simulink model "MotorCtrl_DTC_Math"  (R2023b)
settings: Solver=FixedStepDiscrete  StartTime=0.0  StopTime=5  FixedStep=MC_Sim_BaseStep  RelTol=1e-3  EnableMultiTasking=on
values from neighbouring files (symbols this model uses):
  MC_ADC_BitNum = 0.0    [MotorControlDataDictionary_Math.sldd]
  MC_ADC_Offset = 0.0    [MotorControlDataDictionary_Math.sldd]
  MC_ADC_VRef = 1.0    [MotorControlDataDictionary_Math.sldd]
  MC_Const_DutyL = 0.2    [MotorControlDataDictionary_Math.sldd]
  MC_Const_DutyS = 0.8    [MotorControlDataDictionary_Math.sldd]
  MC_CSA_Gain = 1.0    [MotorControlDataDictionary_Math.sldd]
  MC_Input_Vdc = 13.5    [MotorControlDataDictionary_Math.sldd]
  MC_MOS_DeadTime = 1.0E-6    [MotorControlDataDictionary_Math.sldd]
  MC_Motor_Mechinal_Damp = 1.0E-5    [MotorControlDataDictionary_Math.sldd]
  MC_Motor_Mechinal_Fric = 0.0    [MotorControlDataDictionary_Math.sldd]
  MC_Motor_Mechinal_Inertia = 0.0103    [MotorControlDataDictionary_Math.sldd]
  MC_Motor_Phi = 0.0059190254913385806    [MotorControlDataDictionary_Math.sldd]
  MC_Motor_Rotor_Pn = 4.0    [MotorControlDataDictionary_Math.sldd]
  MC_Motor_Stator_Ld = 5.6345E-5    [MotorControlDataDictionary_Math.sldd]
  MC_Motor_Stator_Lq = 5.6345E-5    [MotorControlDataDictionary_Math.sldd]
  MC_Motor_Stator_Rs = 0.0286    [MotorControlDataDictionary_Math.sldd]
  MC_Param_CurrentPI_Ki = 0.0071879639914134473    [MotorControlDataDictionary_Math.sldd]
  MC_Param_CurrentPI_Kp = 0.283220860906427    [MotorControlDataDictionary_Math.sldd]
  MC_Param_CurrentPI_UdInteMax = 7.794228634059948    [MotorControlDataDictionary_Math.sldd]
  MC_Param_CurrentPI_UdInteMin = -7.794228634059948    [MotorControlDataDictionary_Math.sldd]
  MC_Param_CurrentPI_UdMax = 7.794228634059948    [MotorControlDataDictionary_Math.sldd]
  MC_Param_CurrentPI_UdMin = -7.794228634059948    [MotorControlDataDictionary_Math.sldd]
  MC_Param_CurrentPI_UqInteMax = 7.794228634059948    [MotorControlDataDictionary_Math.sldd]
  MC_Param_CurrentPI_UqInteMin = -7.794228634059948    [MotorControlDataDictionary_Math.sldd]
  MC_Param_CurrentPI_UqMax = 7.794228634059948    [MotorControlDataDictionary_Math.sldd]
  MC_Param_CurrentPI_UqMin = -7.794228634059948    [MotorControlDataDictionary_Math.sldd]
  MC_Param_Flux_Gamma = 750000.0    [MotorControlDataDictionary_Math.sldd]
  MC_Param_Flux_Lalpha = 5.6345E-5    [MotorControlDataDictionary_Math.sldd]
  MC_Param_Flux_Lbeta = 5.6345E-5    [MotorControlDataDictionary_Math.sldd]
  MC_Param_Flux_Ralpha = 0.0286    [MotorControlDataDictionary_Math.sldd]
  MC_Param_Flux_Rbeta = 0.0286    [MotorControlDataDictionary_Math.sldd]
  MC_Param_Luen_BEMFalpha = -17747.803709290976    [MotorControlDataDictionary_Math.sldd]
  MC_Param_Luen_BEMFbeta = -17747.803709290976    [MotorControlDataDictionary_Math.sldd]
  MC_Param_Luen_BEMFErr = -8.0    [MotorControlDataDictionary_Math.sldd]
  MC_Param_Luen_Currentalpha = -507.58718608572195    [MotorControlDataDictionary_Math.sldd]
  MC_Param_Luen_Currentbeta = -507.58718608572195    [MotorControlDataDictionary_Math.sldd]
  MC_Param_Luen_CurrentErr = -8.0    [MotorControlDataDictionary_Math.sldd]
  MC_Param_Luen_PLL_Ki = 2.3480975196640594    [MotorControlDataDictionary_Math.sldd]
  MC_Param_Luen_PLL_Kp = 153.24842212633141    [MotorControlDataDictionary_Math.sldd]
  MC_Param_Luen_Voltagealpha = 17747.803709290976    [MotorControlDataDictionary_Math.sldd]
  MC_Param_Luen_Voltagebeta = 17747.803709290976    [MotorControlDataDictionary_Math.sldd]
  MC_Param_PhasetoReal = 500.0    [MotorControlDataDictionary_Math.sldd]
  MC_Param_SMO_CoffA = 0.97462064069571386    [MotorControlDataDictionary_Math.sldd]
  MC_Param_SMO_CoffB = 0.88739018546454884    [MotorControlDataDictionary_Math.sldd]
  MC_Param_SpeedCtrl_IdMax = 60.0    [MotorControlDataDictionary_Math.sldd]
  MC_Param_SpeedCtrl_IdMin = -60.0    [MotorControlDataDictionary_Math.sldd]
  MC_Param_SpeedCtrl_IqMax = 60.0    [MotorControlDataDictionary_Math.sldd]
  MC_Param_SpeedCtrl_IqMin = -60.0    [MotorControlDataDictionary_Math.sldd]
  MC_Param_SpeedPI_Ki = 0.57248683633241571    [MotorControlDataDictionary_Math.sldd]
  MC_Param_SpeedPI_Kp = 9.1114109857344836    [MotorControlDataDictionary_Math.sldd]
  MC_Param_SpeedtoTheta = 5.0E-5    [MotorControlDataDictionary_Math.sldd]
  MC_Param_SVPWM_DutyMax = 0.98    [MotorControlDataDictionary_Math.sldd]
  MC_Param_SVPWM_DutyMin = 0.02    [MotorControlDataDictionary_Math.sldd]
  MC_Param_SVPWM_SampleOffset1 = 0.02    [MotorControlDataDictionary_Math.sldd]
  MC_Param_SVPWM_SampleOffset2 = 0.015    [MotorControlDataDictionary_Math.sldd]
  MC_Param_SVPWM_SampleValid = 0.011999999999999999    [MotorControlDataDictionary_Math.sldd]
  MC_Sample_CurrentNoise = 1.0E-15    [MotorControlDataDictionary_Math.sldd]
  MC_Sample_Rs = 0.002    [MotorControlDataDictionary_Math.sldd]
  MC_Sample_VbusNoise = 1.0E-15    [MotorControlDataDictionary_Math.sldd]
  MC_Sim_BaseStep = 5.0E-8    [MotorControlDataDictionary_Math.sldd]
  MC_Sim_HFTStep = 5.0E-5    [MotorControlDataDictionary_Math.sldd]
  MC_Sim_MFTStep = 0.002    [MotorControlDataDictionary_Math.sldd]
libraries: simulink x29, spsVoltageMeasurementLib x2, spsDCVoltageSourceLib x1, spsGroundLib x1, spsPermanentMagnetSynchronousMachineLib x1, spsSeriesRLCBranchLib x1, spsThreePhaseVIMeasurementLib x1, spsUniversalBridgeLib x1, sps_lib x1
(part 1 of 5)
settings Model: DataDictionary=MotorControlDataDictionary_Math.sldd  SimulationMode=accelerator  Creator=YXuan  LastModifiedBy=YXuan
settings SolverCC: AutoInsertRateTranBlk=on
settings OptimizationCC: DefaultParameterBehavior=Inlined  DefaultUnderspecifiedDataType=single  EnhancedBackFolding=on  PassReuseOutputArgsAs=Individual arguments  ZeroExternalMemoryAtStartup=off  ZeroInternalMemoryAtStartup=off  EfficientFloat2IntCast=on  OptimizeBlockOrder=speed  DifferentSizesBufferReuse=on  OptimizationCustomize=off  EfficientTunableParamExpr=on
settings DebuggingCC: ParameterPrecisionLossMsg=none
settings ModelReferenceCC: EnableRefExpFcnMdlSchedulingChecks=on
settings SFSimCC: MATLABDynamicMemAlloc=off
settings RTWCC: Description=Embedded Coder  SystemTargetFile=ert.tlc  GenCodeOnly=on  TemplateMakefile=ert_default_tmf  Toolchain=Microsoft Visual C++ 2022 v17.0 | nmake (64-bit Windows)
settings CodeAppCC: ForceParamTrailComments=on  IgnoreCustomStorageClasses=off  IgnoreTestpoints=on  OperatorAnnotations=on  SimulinkDataObjDesc=on  SFDataObjDesc=on  InsertBlockDesc=on
settings ERTTargetCC: TargetLangStandard=C99 (ISO)  InferredTypesCompatibility=on  GenerateSampleERTMain=on  CombineSignalStateStructs=on  SupportAbsoluteTime=off  SupportNonFinite=off  SupportComplex=off  RemoveDisableFunc=on  InlinedParameterPlacement=NonHierarchical  ERTCustomFileTemplate=example_file_process.tlc

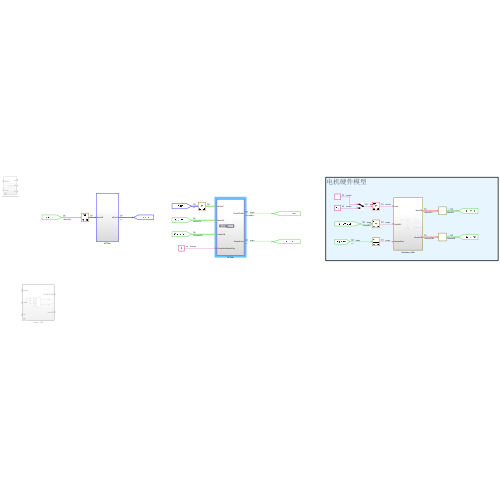
[thumbnail: Simulink's stored preview of the top-level diagram]
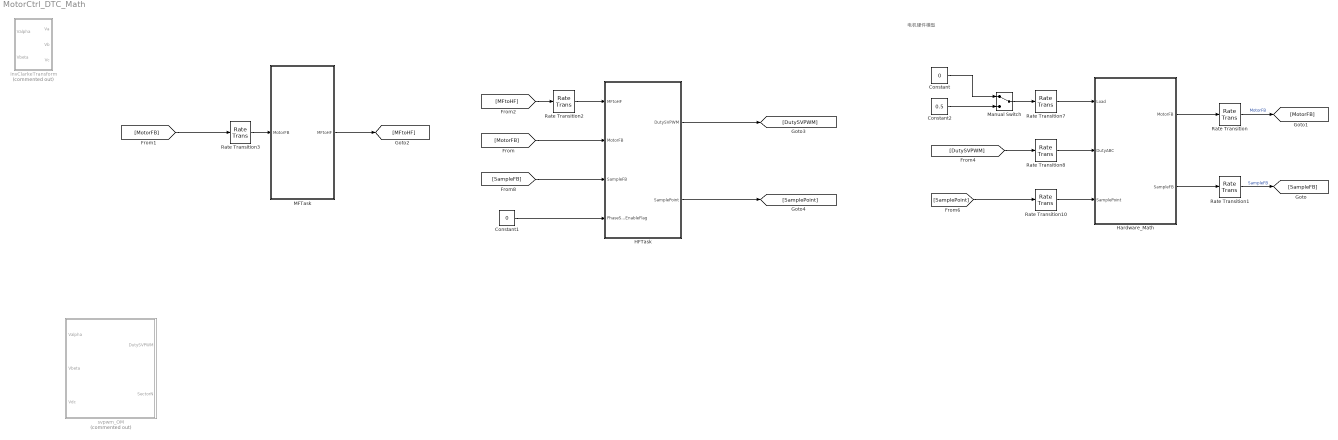
== system MotorCtrl_DTC_Math ==
  note: 电机硬件模型
  Constant : Constant  Value=0
  Constant1 : Constant  Value=0  OutDataTypeStr=boolean
  Constant2 : Constant  Value=0.5
  HFTask : Subsystem  TreatAsAtomicUnit=on  SystemSampleTime=MC_Sim_HFTStep
  Hardware_Math : Subsystem  SystemSampleTime=MC_Sim_BaseStep  VariantControl=MC_Hardware_Motor_Model ==1&MC_Hardware_MotorMOS_Model==1
  MFTask : Subsystem  TreatAsAtomicUnit=on  SystemSampleTime=MC_Sim_MFTStep
  Manual Switch : ManualSwitch
  Rate Transition : RateTransition  OutPortSampleTime=MC_Sim_HFTStep
  Rate Transition1 : RateTransition  OutPortSampleTime=MC_Sim_HFTStep
  Rate Transition10 : RateTransition  OutPortSampleTime=MC_Sim_BaseStep
  Rate Transition2 : RateTransition  OutPortSampleTime=MC_Sim_HFTStep
  Rate Transition3 : RateTransition  OutPortSampleTime=MC_Sim_MFTStep
  Rate Transition7 : RateTransition  OutPortSampleTime=MC_Sim_BaseStep
  Rate Transition8 : RateTransition  OutPortSampleTime=MC_Sim_BaseStep
  invClarkeTransform : Subsystem  Commented=on
  svpwm_OM : Subsystem  Commented=on  TreatAsAtomicUnit=on  SystemSampleTime=MC_Sim_HFTStep
      settings: RTWSystemCode=Nonreusable function  RTWFcnNameOpts=Use subsystem name
  wires:
  Hardware_Math/2(SampleFB) -> Rate Transition1/1
  Rate Transition8/1 -> Hardware_Math/2(DutyABC)
  Hardware_Math/1(MotorFB) -> Rate Transition/1
  [SamplePoint] -> Rate Transition10/1
  [DutySVPWM] -> Rate Transition8/1
  Rate Transition1/1 -> [SampleFB]  "SampleFB"
  Rate Transition10/1 -> Hardware_Math/3(SamplePoint)
  Rate Transition7/1 -> Hardware_Math/1(Load)
  Rate Transition/1 -> [MotorFB]  "MotorFB"
  [MotorFB] -> Rate Transition3/1
  MFTask/1(MFtoHF) -> [MFtoHF]
  [MFtoHF] -> Rate Transition2/1
  Constant1/1 -> HFTask/4(PhaseShortEnableFlag)
  [SampleFB] -> HFTask/3(SampleFB)
  [MotorFB] -> HFTask/2(MotorFB)
  HFTask/1(DutySVPWM) -> [DutySVPWM]
  HFTask/2(SamplePoint) -> [SamplePoint]
  Rate Transition2/1 -> HFTask/1(MFtoHF)
  Rate Transition3/1 -> MFTask/1(MotorFB)
  Manual Switch/1 -> Rate Transition7/1
  Constant/1 -> Manual Switch/1
  Constant2/1 -> Manual Switch/2

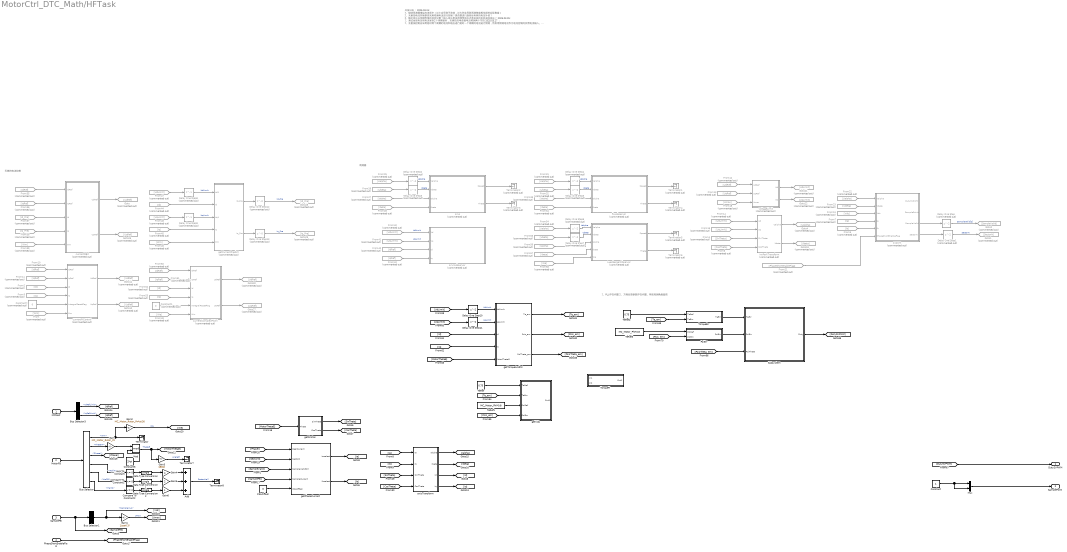
== system MotorCtrl_DTC_Math/HFTask ==
  note: 1、PLL存在问题
      | 2、方程反馈参数存在问题，导致观测角度超前
  note: 观测器
  note: 无差拍电流控制
  note: 开发日志：
      | 2025.03.24:
      | 1、磁链观测器增益应该适中（过小会导致不收敛，过大则会导致观测角度相位超前实际角度）
      | 2、无差拍电流控制是否采用预测电流进行控制？是否要进行旋转反电势的电压补偿？
      | 3、静态电压补偿模型增益如何设置？输入电压是采用理想电压还是采样的电机实际电压？
      | 2025.03.25:
      | 1、测试发现电压和电流呈现2个周期延时，无差拍应考虑做电流预测两个节拍
      | 2025.03.27：
      | 1、无差拍控制应采用延时两个周期的电流和电压进行延时一个周期的电流进行预测，然后用预测电流作为电流控制的反馈电流输入。
      | 2025.07.08：
      | 1、取消FOC控制相关的电流控制环路和SVPWM模块
      | 2、增加电机定子磁链估算模块
      | 3、增加传统DTC控制相关的逆变器开关表
  MFtoHF : Inport
  MotorFB : Inport  Port=2
  SampleFB : Inport  Port=3
  PhaseShortEnableFlag : Inport  Port=4
  Add : Sum  Inputs=+++
  Bus Selector : BusSelector  OutputSignals=Wm,ThetaM,PhaseI,HallA,HallB,HallC
  Bus Selector1 : BusSelector  OutputSignals=SampleVus
  Bus Selector3 : BusSelector  OutputSignals=IdRefLimit,IqRefLimit
  CSAOffset : Constant  Value=0  OutDataTypeStr=single
  Compare To Constant : simulink/Logic and Bit Operations/Compare To Constant  relop=<=  const=0  OutDataTypeStr=boolean
  Compare To Constant1 : simulink/Logic and Bit Operations/Compare To Constant  relop=<=  const=0  OutDataTypeStr=boolean
  Compare To Constant2 : simulink/Logic and Bit Operations/Compare To Constant  relop=<=  const=0  OutDataTypeStr=boolean
  Constant : Constant  OutDataTypeStr=single
  Constant1 : Constant  Commented=on  Value=0  OutDataTypeStr=boolean
  Constant2 : Constant  Commented=on  Value=0  OutDataTypeStr=boolean
  Constant6 : Constant  Value=2*pi  OutDataTypeStr=single
  Data Type Conversion : DataTypeConversion  OutDataTypeStr=single  RndMeth=Simplest  SaturateOnIntegerOverflow=off
  Data Type Conversion1 : DataTypeConversion  OutDataTypeStr=single  RndMeth=Simplest  SaturateOnIntegerOverflow=off
  Data Type Conversion2 : DataTypeConversion  OutDataTypeStr=single  RndMeth=Simplest  SaturateOnIntegerOverflow=off
  Delay One Step{,1..7} (8 alike) : Delay  Commented=on
  Delay One Step10 : Delay
  Delay One Step11 : Delay
  Delay One Step12 : Delay  Commented=on  DelayLength=0
  Delay One Step13 : Delay  Commented=on  DelayLength=0
  Delay One Step8 : Delay  Commented=on  DelayLength=1
  Delay One Step9 : Delay  Commented=on  DelayLength=1
  From : From  Commented=on  GotoTag=Wm
  From{10,35,42,50} (4 alike) : From  Commented=on  GotoTag=IdRef
  From{11,36,43,51} (4 alike) : From  Commented=on  GotoTag=IqRef
  From12 : From  Commented=on  GotoTag=UdRef
  From13 : From  Commented=on  GotoTag=UqRef
  From14 : From  Commented=on  GotoTag=UdLimit
  From15 : From  Commented=on  GotoTag=UqLimit
  From18 : From  Commented=on  GotoTag=Umax
  From2 : From  Commented=on  GotoTag=Id
  From21 : From  Commented=on  GotoTag=PhaseShortEnableFlag
  From{22,25,31,54} (4 alike) : From  Commented=on  GotoTag=Ualpha
  From{23,26,32,55} (4 alike) : From  Commented=on  GotoTag=Ubeta
  From24 : From  Commented=on  GotoTag=Vdc
  From27 : From  Commented=on  GotoTag=Ialpha
  From28 : From  Commented=on  GotoTag=Ibeta
  From3 : From  Commented=on  GotoTag=Iq
  From33 : From  Commented=on  GotoTag=Ialpha
  From34 : From  Commented=on  GotoTag=Ibeta
  From37 : From  Commented=on  GotoTag=Id_Pre
  From38 : From  Commented=on  GotoTag=Iq_Pre
  From39 : From  Commented=on  GotoTag=Wm
  From4 : From  Commented=on  GotoTag=SinTheta
  From40 : From  Commented=on  GotoTag=UdLimit
  From41 : From  Commented=on  GotoTag=UqLimit
  From44 : From  Commented=on  GotoTag=Id
  From45 : From  Commented=on  GotoTag=Iq
  From46 : From  Commented=on  GotoTag=Wm
  From47 : From  Commented=on  GotoTag=UdLimit
  From48 : From  Commented=on  GotoTag=UqLimit
  From49 : From  Commented=on  GotoTag=We
  From5 : From  Commented=on  GotoTag=Ib
  From52 : From  Commented=on  GotoTag=Id
  From53 : From  Commented=on  GotoTag=Iq
  From56 : From  Commented=on  GotoTag=Ialpha
  From57 : From  Commented=on  GotoTag=Ibeta
  From58 : From  Commented=on  GotoTag=We
  From6 : From  Commented=on  GotoTag=CosTheta
  From7 : From  Commented=on  GotoTag=Ia
  Gain : Gain  Gain=MC_Motor_Rotor_Pn  OutDataTypeStr=single
  Gain1 : Gain  Gain=1/sqrt(3)  OutDataTypeStr=single
  Gain2 : Gain  Gain=MC_Motor_Rotor_Pn*pi/30
  Gain3 : Gain  Gain=180/pi
  Gain4 : Gain  Gain=4
  Gain5 : Gain  Gain=2
  Gain6 : Gain
  Goto : Goto  Commented=on  GotoTag=UdRef
  Goto1 : Goto  Commented=on  GotoTag=SectorN
  Goto10 : Goto  Commented=on  GotoTag=UqRef
  Goto14 : Goto  Commented=on  GotoTag=UdRef
  Goto18 : Goto  Commented=on  GotoTag=Ubeta
  Goto2 : Goto  Commented=on  GotoTag=SampleValid
  Goto21 : Goto  Commented=on  GotoTag=UdLimit
  Goto22 : Goto  Commented=on  GotoTag=UqLimit
  Goto26 : Goto  Commented=on  GotoTag=UqRef
  Goto27 : Goto  Commented=on  GotoTag=UqRef
  Goto28 : Goto  Commented=on  GotoTag=Id_Pre
  Goto29 : Goto  Commented=on  GotoTag=Iq_Pre
  Goto30 : Goto  Commented=on  GotoTag=UdRef
  Goto4 : Goto  Commented=on  GotoTag=Ualpha
  LuenbergerObservor : Subsystem  Commented=on
  Mod : Math  Operator=mod
  Mux : Mux  Inputs=2
  PsiErr : Subsystem
  Subsystem : Subsystem
  TeRef : Constant  Value=0.75  OutDataTypeStr=single
  TeRef1 : Constant  Value=MC_Motor_Phi*0.8  OutDataTypeStr=single
  TeRef2 : Constant  Value=0.75  OutDataTypeStr=single
  TeRef3 : Constant  Value=MC_Motor_Phi*0.8  OutDataTypeStr=single
  Terminator : Terminator
  Terminator{1..6} (6 alike) : Terminator  Commented=on
  Terminator7 : Terminator
  Terminator8 : Terminator
  TorqueErr : Subsystem
  TorquePI : Subsystem
  axisTransform : Subsystem
  currentComplexPICtrl : Subsystem  Commented=on
  currentDBC : Subsystem  Commented=on
  currentPIControl : Subsystem  Commented=on
  fluxobservor : Subsystem  Commented=on
  getCurrentPredict : Subsystem  Commented=on
  getPhaseCurrent : Subsystem
  getSinCos : Subsystem
  getTorqueAndPsi : Subsystem
  getVdq : Subsystem
  invParkTransform : Subsystem  Commented=on
  scvmobservor : Subsystem  Commented=on
  smo : Subsystem  Commented=on
  svpwm : Subsystem  Commented=on  TreatAsAtomicUnit=on
  voltageLimit : Subsystem  Commented=on
  DutySVPWM : Outport
  SamplePoint : Outport  Port=2
  wires:
  MFtoHF/1 -> Bus Selector3/1
  Delay One Step2/1 -> smo/1(Valpha)  "Ualpha"
  From25/1 -> Delay One Step2/1
  Delay One Step3/1 -> smo/2(Vbeta)  "Ubeta"
  From26/1 -> Delay One Step3/1
  From27/1 -> smo/3(Ialpha)
  From28/1 -> smo/4(Ibeta)
  smo/1(Speed) -> Terminator2/1
  smo/2(Theta) -> Terminator3/1
  From21/1 -> svpwm/6(PhaseShortEnableFlag)
  From18/1 -> voltageLimit/3(Umax)
  svpwm/4(SectorN) -> Delay One Step1/1
  axisTransform/2(Ibeta) -> [Ibeta]
  svpwm/3(SampleValid) -> Delay One Step/1
  [SampleFB] -> getPhaseCurrent/4(SampleCurrent)
  [SectorN] -> getPhaseCurrent/2(SectorN)
  From12/1 -> voltageLimit/1(UdRef)
  From14/1 -> invParkTransform/1(Ud)
  currentPIControl/1(UdRef) -> Goto14/1
  From23/1 -> svpwm/2(Vbeta)
  axisTransform/1(Ialpha) -> [Ialpha]
  From13/1 -> voltageLimit/2(UqRef)
  From22/1 -> svpwm/1(Valpha)
  [Ia] -> axisTransform/1(Ia)
  currentPIControl/2(UqRef) -> Goto10/1
  From24/1 -> svpwm/3(Vdc)
  voltageLimit/1(Ud) -> Goto21/1
  [MotorThetaE] -> getSinCos/1(Theta)
  From2/1 -> currentPIControl/3(Id)
  getSinCos/1(SinTheta) -> [SinTheta]
  [SampleValid] -> getPhaseCurrent/3(SampleValid[2])
  axisTransform/3(Id) -> [Id]
  getPhaseCurrent/2(Ibselect) -> [Ib]
  From/1 -> currentPIControl/6(Wm)
  axisTransform/4(Iq) -> [Iq]
  From3/1 -> currentPIControl/4(Iq)
  Constant2/1 -> currentPIControl/5(IntregralResetFlag)
  [Ib] -> axisTransform/2(Ib)
  From15/1 -> invParkTransform/2(Uq)
  From4/1 -> invParkTransform/3(SinTheta)
  Delay One Step1/1 -> Goto1/1  "SectorN"
  From6/1 -> invParkTransform/4(CosTheta)
  [PhaseI] -> getPhaseCurrent/1(RealCurrent)
  invParkTransform/1(Ualpha) -> Goto4/1
  Delay One Step/1 -> Goto2/1  "SampleValid[2]"
  getSinCos/2(CosTheta) -> [CosTheta]
  voltageLimit/2(Uq) -> Goto22/1
  [SinTheta] -> axisTransform/3(SinTheta)
  getPhaseCurrent/1(Iaselect) -> [Ia]
  CSAOffset/1 -> getPhaseCurrent/5(CSAOffset)
  [CosTheta] -> axisTransform/4(CosTheta)
  invParkTransform/2(Ubeta) -> Goto18/1
  From5/1 -> svpwm/5(Ib)
  From7/1 -> svpwm/4(Ia)
  Bus Selector/2 -> Gain/1  "<ThetaM>"
  PhaseShortEnableFlag/1 -> [PhaseShortEnableFlag]
  Bus Selector/1 -> Terminator/1, Gain2/1  "<Wm>"
  Mod/1 -> Gain3/1, [MotorThetaE]  "ThetaE"
  Bus Selector/3 -> [PhaseI]  "<PhaseI>"
  Gain/1 -> Mod/1
  Bus Selector1/1 -> [Vdc], Gain1/1  "<SampleVus>"
  SampleFB/1 -> [SampleFB], Bus Selector1/1
  Gain1/1 -> [Umax]  "Umax"
  Constant6/1 -> Mod/2
  MotorFB/1 -> Bus Selector/1
  Bus Selector3/1 -> [IdRef]  "<IdRefLimit>"
  Bus Selector3/2 -> [IqRef]  "<IqRefLimit>"
  From10/1 -> currentPIControl/1(IdRef)
  From11/1 -> currentPIControl/2(IqRef)
  From34/1 -> fluxobservor/4(Ibeta)
  From33/1 -> fluxobservor/3(Ialpha)
  From32/1 -> Delay One Step5/1
  From31/1 -> Delay One Step4/1
  Delay One Step4/1 -> fluxobservor/1(Valpha)  "Ualpha"
  Delay One Step5/1 -> fluxobservor/2(Vbeta)  "Ubeta"
  fluxobservor/1(Speed) -> Terminator1/1
  fluxobservor/2(Theta) -> Terminator4/1
  currentDBC/2(UqRef) -> Goto26/1
  From36/1 -> currentDBC/2(IqRef)
  From35/1 -> currentDBC/1(IdRef)
  From37/1 -> currentDBC/3(Id)
  From38/1 -> currentDBC/4(Iq)
  From39/1 -> currentDBC/5(Wm)
  From41/1 -> scvmobservor/2(Vq)  "UqLimit"
  From40/1 -> scvmobservor/1(Vd)  "UdLimit"
  From42/1 -> scvmobservor/3(Id)
  From43/1 -> scvmobservor/4(Iq)
  Gain2/1 -> [We]  "We"
  From44/1 -> getCurrentPredict/2(Id)
  From45/1 -> getCurrentPredict/4(Iq)
  From46/1 -> getCurrentPredict/5(Wm)
  From47/1 -> Delay One Step8/1
  From48/1 -> Delay One Step9/1
  getCurrentPredict/1(Id_Pre) -> Delay One Step12/1
  getCurrentPredict/2(Iq_Pre) -> Delay One Step13/1
  currentDBC/1(UdRef) -> Goto/1
  Delay One Step8/1 -> getCurrentPredict/1(Ud1)  "UdLimit"
  Delay One Step9/1 -> getCurrentPredict/3(Uq1)  "UqLimit"
  Delay One Step12/1 -> Goto28/1  "Id_Pre"
  Delay One Step13/1 -> Goto29/1  "Iq_Pre"
  From51/1 -> currentComplexPICtrl/2(IqRef)
  From50/1 -> currentComplexPICtrl/1(IdRef)
  Constant1/1 -> currentComplexPICtrl/5(IntregralResetFlag)
  From53/1 -> currentComplexPICtrl/4(Iq)
  From49/1 -> currentComplexPICtrl/6(Wm)
  From52/1 -> currentComplexPICtrl/3(Id)
  currentComplexPICtrl/2(UqRef) -> Goto27/1
  currentComplexPICtrl/1(UdRef) -> Goto30/1
  LuenbergerObservor/1(Speed) -> Terminator5/1
  LuenbergerObservor/2(Theta) -> Terminator6/1
  From57/1 -> LuenbergerObservor/4(Ibeta)
  From56/1 -> LuenbergerObservor/3(Ialpha)
  From55/1 -> Delay One Step7/1
  From54/1 -> Delay One Step6/1
  Delay One Step7/1 -> LuenbergerObservor/2(Vbeta)  "Ubeta"
  Delay One Step6/1 -> LuenbergerObservor/1(Valpha)  "Ualpha"
  From58/1 -> LuenbergerObservor/5(We)
  Delay One Step11/1 -> getTorqueAndPsi/2(UqLimit)  "UqLimit"
  Delay One Step10/1 -> getTorqueAndPsi/1(UdLimit)  "UdLimit"
  [Id] -> getTorqueAndPsi/3(Id)
  [Iq] -> getTorqueAndPsi/4(Iq)
  [UdLimit] -> Delay One Step10/1
  [UqLimit] -> Delay One Step11/1
  Gain3/1 -> Terminator7/1  "AngleE"
  Bus Selector/4 -> Compare To Constant/1  "<HallA>"
  Bus Selector/5 -> Compare To Constant1/1  "<HallB>"
  Bus Selector/6 -> Compare To Constant2/1  "<HallC>"
  Compare To Constant/1 -> Data Type Conversion/1
  Compare To Constant1/1 -> Data Type Conversion1/1
  Compare To Constant2/1 -> Data Type Conversion2/1
  Data Type Conversion/1 -> Gain4/1
  Data Type Conversion1/1 -> Gain5/1
  Data Type Conversion2/1 -> Gain6/1
  Gain4/1 -> Add/1
  Gain5/1 -> Add/2
  Gain6/1 -> Add/3
  Add/1 -> Terminator8/1  "SectorHall"
  getTorqueAndPsi/2(Psis_em) -> [Psis_em]
  getTorqueAndPsi/3(PsiTheta_em) -> [PsisTheta_em]
  [MotorThetaE] -> getTorqueAndPsi/5("MotorThetaE ")
  getTorqueAndPsi/1(Te_em) -> [Te_em]
  [Psis_em] -> getVdq/4(PsiEm)
  TeRef1/1 -> getVdq/3(PsiRef)
  Mux/1 -> SamplePoint/1
  Constant/1 -> Mux/2, Mux/1
  [PsisTheta_em] -> Subsystem/3(PsiTheta)
  TeRef3/1 -> PsiErr/1(PsiRef)
  [Psis_em] -> PsiErr/2(PsiEm)
  [Te_em] -> TorqueErr/2(TeEm)
  TeRef2/1 -> TorqueErr/1(TeRef)
  TorqueErr/1(TeErr) -> Subsystem/1(TeErr)
  PsiErr/1(PsiErr) -> Subsystem/2(PsiErr)
  [DutySVPWM] -> DutySVPWM/1
  Subsystem/1(Duty) -> [DutySVPWM]
  TeRef/1 -> getVdq/1(TeRef)
  [Te_em] -> getVdq/2(TeEm)

== system MotorCtrl_DTC_Math/Hardware_Math ==
  Load : Inport
  DutyABC : Inport  Port=2
  SamplePoint : Inport  Port=3
  Add : Sum
  Add1 : Sum
  Add2 : Sum
  AngleProcess : Subsystem
  Band-Limited White Noise : simulink/Sources/Band-Limited White Noise  Cov=[MC_Sample_CurrentNoise]  Ts=MC_Sim_BaseStep  seed=[23341]
  Band-Limited White Noise1 : simulink/Sources/Band-Limited White Noise  Cov=[MC_Sample_VbusNoise]  Ts=MC_Sim_BaseStep  seed=[23341]
  Bus Creator : BusCreator  Inputs=8
  Bus Creator1 : BusCreator  Inputs=2
  Bus Selector : BusSelector  OutputSignals=Rotor angle thetam (rad),Rotor speed wm (rad/s),Electromagnetic torque Te (N*m),Hall effect signal h_a,Hall effect signal h_b,Hall effect signal h_c
  Data Type Conversion{,1..6} (7 alike) : DataTypeConversion  OutDataTypeStr=single  SaturateOnIntegerOverflow=off  RndMeth=Floor
  Gain : Gain  Gain=0.000154
  Gain1 : Gain  Gain=30/pi
  MotorHardware : Subsystem
  PWMGenerate : Subsystem  SystemSampleTime=MC_Sim_BaseStep
  VbusSample : Subsystem
  currentSample : Subsystem  Variant=on  VariantControl=Subsystem
  MotorFB : Outport
  SampleFB : Outport  Port=2
  wires:
  Band-Limited White Noise/1 -> Add/2
  Add/1 -> currentSample/2(Current)
  Add1/1 -> VbusSample/1(Vbus)
  Band-Limited White Noise1/1 -> Add1/2
  [CurrentSampleTrigger] -> currentSample/1(SampleTrigger)
  PWMGenerate/2(CurrentSamplTrigger) -> [CurrentSampleTrigger]
  Bus Selector/2 -> Gain1/1  "<Rotor speed wm (rad/s)>"
  DutyABC/1 -> PWMGenerate/1(DutyABC)
  Bus Selector/1 -> AngleProcess/1(In1)  "<Rotor angle thetam (rad)>"
  SamplePoint/1 -> PWMGenerate/2(SamplePoint)
  Bus Selector/3 -> Data Type Conversion1/1  "<Electromagnetic torque Te (N*m)>"
  Load/1 -> [Load_Input]
  Gain1/1 -> Data Type Conversion/1, [Wm]
  AngleProcess/1(Out1) -> Bus Creator/1
  [PhaseV] -> Data Type Conversion2/1
  [PhaseI] -> Data Type Conversion3/1
  VbusSample/1(VbusSample) -> Bus Creator1/1  "SampleVus"
  currentSample/1(SampleCurrent) -> Bus Creator1/2
  Bus Creator1/1 -> SampleFB/1  "SampleFB"
  PWMGenerate/1(Gate) -> MotorHardware/2(PWM)  "PWM"
  MotorHardware/1(Vabc) -> [PhaseV]
  MotorHardware/2(Iabc) -> [PhaseI]
  MotorHardware/3(m) -> Bus Selector/1
  MotorHardware/5(Current) -> Add/1
  MotorHardware/4(Vbus) -> Add1/1
  Data Type Conversion/1 -> Bus Creator/2  "Wm"
  Data Type Conversion1/1 -> Bus Creator/3  "Te"
  Data Type Conversion2/1 -> Bus Creator/7  "PhaseV"
  Data Type Conversion3/1 -> Bus Creator/8  "PhaseI"
  Bus Creator/1 -> MotorFB/1  "MotorFB"
  Add2/1 -> MotorHardware/1(mec)
  [Load_Input] -> Add2/2
  [Wm] -> Gain/1
  Gain/1 -> Add2/1
  Bus Selector/4 -> Data Type Conversion4/1  "<Hall effect signal h_a>"
  Bus Selector/5 -> Data Type Conversion5/1  "<Hall effect signal h_b>"
  Bus Selector/6 -> Data Type Conversion6/1  "<Hall effect signal h_c>"
  Data Type Conversion4/1 -> Bus Creator/4  "HallA"
  Data Type Conversion5/1 -> Bus Creator/5  "HallB"
  Data Type Conversion6/1 -> Bus Creator/6  "HallC"

== system MotorCtrl_DTC_Math/MFTask ==
  MotorFB : Inport
  Bus Creator : BusCreator  Inputs=2
  Bus Selector : BusSelector  OutputSignals=Wm
  Constant : Constant  Value=1500  OutDataTypeStr=single
  From2 : From  Commented=on  GotoTag=SpeedTarget
  From3 : From  Commented=on  GotoTag=SpeedMotor
  Goto : Goto  Commented=on  GotoTag=IdRef
  Goto1 : Goto  Commented=on  GotoTag=IqRef
  getCurrentLimit : Subsystem
  piofSpeed : Subsystem
  smcofSpeed : Subsystem  Commented=on
  MFtoHF : Outport
  wires:
  MotorFB/1 -> Bus Selector/1
  Bus Selector/1 -> [SpeedMotor]  "<Wm>"
  Bus Creator/1 -> MFtoHF/1
  smcofSpeed/1(IdRef) -> Goto/1
  smcofSpeed/2(IqRef) -> Goto1/1
  piofSpeed/1(IdRef) -> [IdRef]
  piofSpeed/2(IqRef) -> [IqRef]
  getCurrentLimit/2(IqRefLimit) -> [IqRefLimit]
  getCurrentLimit/1(IdRefLimit) -> [IdRefLimit]
  [IdRefLimit] -> Bus Creator/1
  [IqRefLimit] -> Bus Creator/2
  Constant/1 -> [SpeedTarget]  "SpeedTarget"
  From2/1 -> smcofSpeed/1(SpeedTarget)
  From3/1 -> smcofSpeed/2(SpeedReal)
  [IdRef] -> getCurrentLimit/1(IdRef)
  [IqRef] -> getCurrentLimit/2(IqRef)
  [SpeedTarget] -> piofSpeed/1(SpeedTarget)
  [SpeedMotor] -> piofSpeed/2(SpeedReal)

== system MotorCtrl_DTC_Math/invClarkeTransform ==
  Valpha : Inport
  Vbeta : Inport  Port=2
  Add : Sum
  Gain : Gain  Gain=-1/2
  Gain1 : Gain  Gain=sqrt(3)/2
  Subtract : Sum  Inputs=+-
  Va : Outport
  Vb : Outport  Port=2
  Vc : Outport  Port=3
  wires:
  Valpha/1 -> Gain/1, Va/1  "Va"
  Vbeta/1 -> Gain1/1
  Gain/1 -> Subtract/1, Add/1
  Gain1/1 -> Subtract/2, Add/2
  Add/1 -> Vb/1  "Vb"
  Subtract/1 -> Vc/1  "Vc"

== system MotorCtrl_DTC_Math/svpwm_OM ==
  Valpha : Inport
  Vbeta : Inport  Port=2
  Vdc : Inport  Port=3
  getVoltageExchange : Subsystem
  setDTCompelte : Subsystem
  DutySVPWM : Outport
  SectorN : Outport  Port=2
  wires:
  getVoltageExchange/4(Vmed) -> setDTCompelte/4(Vmed)
  getVoltageExchange/3(Vc) -> setDTCompelte/3(Vc)
  getVoltageExchange/2(Vb) -> setDTCompelte/2(Vb)
  getVoltageExchange/1(Va) -> setDTCompelte/1(Va)
  Vdc/1 -> getVoltageExchange/3(Vdc)
  Vbeta/1 -> getVoltageExchange/2(Vbeta)
  Valpha/1 -> getVoltageExchange/1(Valpha)
  setDTCompelte/2(DutyABC) -> DutySVPWM/1
  setDTCompelte/1(SectorN) -> SectorN/1

== system MotorCtrl_DTC_Math/HFTask/LuenbergerObservor ==
  Valpha : Inport
  Vbeta : Inport  Port=2
  Ialpha : Inport  Port=3
  Ibeta : Inport  Port=4
  We : Inport  Port=5
  Delay One Step : Delay  DelayLength=1  InitialCondition=single(0)
  Terminator : Terminator
  getE : Subsystem
  getSpeedandTheta : Subsystem
  Speed : Outport
  Theta : Outport  Port=2
  wires:
  getSpeedandTheta/2(Theta) -> Theta/1
  getSpeedandTheta/1(Speed) -> Speed/1
  getE/2(Ebeta) -> getSpeedandTheta/2(Ebeta)
  getE/1(Ealpha) -> getSpeedandTheta/1(Ealpha)
  Ibeta/1 -> getE/4(Ibeta)
  Ialpha/1 -> getE/3(Ialpha)
  Vbeta/1 -> getE/2(Vbeta)
  Valpha/1 -> getE/1(Valpha)
  getSpeedandTheta/3(We) -> Delay One Step/1
  We/1 -> Terminator/1
  Delay One Step/1 -> getE/5(We)

== system MotorCtrl_DTC_Math/HFTask/PsiErr ==
  PsiRef : Inport
  PsiEm : Inport  Port=2
  Subtract : Sum  Inputs=+-
  PsiErr : Outport
  wires:
  Subtract/1 -> PsiErr/1
  PsiRef/1 -> Subtract/1
  PsiEm/1 -> Subtract/2

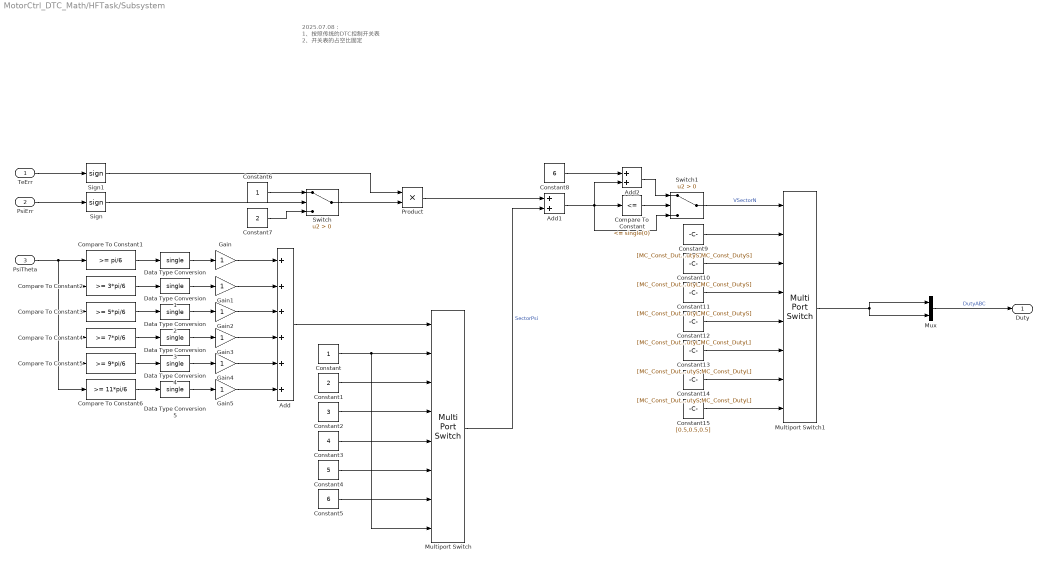
== system MotorCtrl_DTC_Math/HFTask/Subsystem ==
  note: 2025.07.08：
      | 1、按照传统的DTC控制开关表
      | 2、开关表的占空比固定
  TeErr : Inport
  PsiErr : Inport  Port=2
  PsiTheta : Inport  Port=3
  Add : Sum  Inputs=++++++
  Add1 : Sum
  Add2 : Sum
  Compare To Constant : simulink/Logic and Bit Operations/Compare To Constant  relop=<=  const=single(0)  OutDataTypeStr=boolean
  Compare To Constant1 : simulink/Logic and Bit Operations/Compare To Constant  relop=>=  const=pi/6  OutDataTypeStr=boolean
  Compare To Constant2 : simulink/Logic and Bit Operations/Compare To Constant  relop=>=  const=3*pi/6  OutDataTypeStr=boolean
  Compare To Constant3 : simulink/Logic and Bit Operations/Compare To Constant  relop=>=  const=5*pi/6  OutDataTypeStr=boolean
  Compare To Constant4 : simulink/Logic and Bit Operations/Compare To Constant  relop=>=  const=7*pi/6  OutDataTypeStr=boolean
  Compare To Constant5 : simulink/Logic and Bit Operations/Compare To Constant  relop=>=  const=9*pi/6  OutDataTypeStr=boolean
  Compare To Constant6 : simulink/Logic and Bit Operations/Compare To Constant  relop=>=  const=11*pi/6  OutDataTypeStr=boolean
  Constant : Constant  OutDataTypeStr=single
  Constant1 : Constant  Value=2  OutDataTypeStr=single
  Constant10 : Constant  Value=[MC_Const_DutyL,MC_Const_DutyL,MC_Const_DutyS]  OutDataTypeStr=single
  Constant11 : Constant  Value=[MC_Const_DutyS,MC_Const_DutyL,MC_Const_DutyS]  OutDataTypeStr=single
  Constant12 : Constant  Value=[MC_Const_DutyS,MC_Const_DutyL,MC_Const_DutyL]  OutDataTypeStr=single
  Constant13 : Constant  Value=[MC_Const_DutyS,MC_Const_DutyS,MC_Const_DutyL]  OutDataTypeStr=single
  Constant14 : Constant  Value=[MC_Const_DutyL,MC_Const_DutyS,MC_Const_DutyL]  OutDataTypeStr=single
  Constant15 : Constant  Value=[0.5,0.5,0.5]  OutDataTypeStr=single
  Constant2 : Constant  Value=3  OutDataTypeStr=single
  Constant3 : Constant  Value=4  OutDataTypeStr=single
  Constant4 : Constant  Value=5  OutDataTypeStr=single
  Constant5 : Constant  Value=6  OutDataTypeStr=single
  Constant6 : Constant  OutDataTypeStr=single
  Constant7 : Constant  Value=2  OutDataTypeStr=single
  Constant8 : Constant  Value=6  OutDataTypeStr=single
  Constant9 : Constant  Value=[MC_Const_DutyL,MC_Const_DutyS,MC_Const_DutyS]  OutDataTypeStr=single
  Data Type Conversion{,1..5} (6 alike) : DataTypeConversion  OutDataTypeStr=single  RndMeth=Simplest  SaturateOnIntegerOverflow=off
  Gain{,1..5} (6 alike) : Gain
  Multiport Switch : MultiPortSwitch  DataPortOrder=Zero-based contiguous  Inputs=6  DataPortForDefault=Additional data port  zeroidx=on  SaturateOnIntegerOverflow=off  InputSameDT=off
  Multiport Switch1 : MultiPortSwitch  Inputs=6  DataPortForDefault=Additional data port  SaturateOnIntegerOverflow=off  InputSameDT=off
  Mux : Mux  Inputs=2
  Product : Product
  Sign : Signum
  Sign1 : Signum
  Switch : Switch  Criteria=u2 > Threshold  SaturateOnIntegerOverflow=off  InputSameDT=off
  Switch1 : Switch  Criteria=u2 > Threshold  SaturateOnIntegerOverflow=off  InputSameDT=off
  Duty : Outport
  wires:
  PsiErr/1 -> Sign/1
  TeErr/1 -> Sign1/1
  PsiTheta/1 -> Compare To Constant2/1, Compare To Constant3/1, Compare To Constant6/1, Compare To Constant5/1, Compare To Constant4/1, Compare To Constant1/1
  Compare To Constant1/1 -> Data Type Conversion/1
  Compare To Constant2/1 -> Data Type Conversion1/1
  Compare To Constant3/1 -> Data Type Conversion2/1
  Compare To Constant4/1 -> Data Type Conversion3/1
  Compare To Constant5/1 -> Data Type Conversion4/1
  Compare To Constant6/1 -> Data Type Conversion5/1
  Data Type Conversion/1 -> Gain/1
  Data Type Conversion1/1 -> Gain1/1
  Data Type Conversion2/1 -> Gain2/1
  Data Type Conversion3/1 -> Gain3/1
  Data Type Conversion4/1 -> Gain4/1
  Data Type Conversion5/1 -> Gain5/1
  Gain/1 -> Add/1
  Gain1/1 -> Add/2
  Gain2/1 -> Add/3
  Gain3/1 -> Add/4
  Gain4/1 -> Add/5
  Gain5/1 -> Add/6
  Add/1 -> Multiport Switch/1
  Constant/1 -> Multiport Switch/8, Multiport Switch/2
  Constant1/1 -> Multiport Switch/3
  Constant2/1 -> Multiport Switch/4
  Constant3/1 -> Multiport Switch/5
  Constant4/1 -> Multiport Switch/6
  Constant5/1 -> Multiport Switch/7
  Multiport Switch/1 -> Add1/2  "SectorPsi"
  Sign1/1 -> Product/1
  Sign/1 -> Switch/2
  Constant6/1 -> Switch/1
  Constant7/1 -> Switch/3
  Switch/1 -> Product/2
  Product/1 -> Add1/1
  Add1/1 -> Add2/2, Switch1/3, Compare To Constant/1
  Compare To Constant/1 -> Switch1/2
  Add2/1 -> Switch1/1
  Constant8/1 -> Add2/1
  Switch1/1 -> Multiport Switch1/1  "VSectorN"
  Constant9/1 -> Multiport Switch1/2
  Constant10/1 -> Multiport Switch1/3
  Constant11/1 -> Multiport Switch1/4
  Constant12/1 -> Multiport Switch1/5
  Constant13/1 -> Multiport Switch1/6
  Constant14/1 -> Multiport Switch1/7
  Constant15/1 -> Multiport Switch1/8
  Mux/1 -> Duty/1  "DutyABC"
  Multiport Switch1/1 -> Mux/1, Mux/2

== system MotorCtrl_DTC_Math/HFTask/TorqueErr ==
  TeRef : Inport
  TeEm : Inport  Port=2
  Subtract : Sum  Inputs=+-
  TeErr : Outport
  wires:
  TeEm/1 -> Subtract/2
  TeRef/1 -> Subtract/1
  Subtract/1 -> TeErr/1

== system MotorCtrl_DTC_Math/HFTask/TorquePI ==
  In1 : Inport
  In2 : Inport  Port=2
  Add1 : Sum
  Add2 : Sum
  Delay One Step14 : Delay  DelayLength=1
  Gain7 : Gain  Gain=0.1
  Gain8 : Gain  Gain=0.1*MC_Sim_HFTStep
  Subtract : Sum  Inputs=+-
  Out1 : Outport
  wires:
  Delay One Step14/1 -> Add1/2
  Add2/1 -> Out1/1
  Add1/1 -> Add2/2, Delay One Step14/1
  Gain8/1 -> Add1/1
  Gain7/1 -> Add2/1
  Subtract/1 -> Gain8/1, Gain7/1
  In1/1 -> Subtract/1
  In2/1 -> Subtract/2

== system MotorCtrl_DTC_Math/HFTask/axisTransform ==
  Ia : Inport
  Ib : Inport  Port=2
  SinTheta : Inport  Port=3
  CosTheta : Inport  Port=4
  Add1 : Sum
  Product{,1..3} (4 alike) : Product
  Signal Copy : SignalConversion  OverrideOpt=off
  Subtract : Sum  Inputs=-+
  a_plus_2b : Sum  Inputs=+++  RndMeth=Simplest  OutDataTypeStr=Inherit: Same as first input
  one_by_sqrt3 : Gain  Gain=1/sqrt(3)  RndMeth=Simplest  OutDataTypeStr=Inherit: Same as input
  Ialpha : Outport
  Ibeta : Outport  Port=2
  Id : Outport  Port=3
  Iq : Outport  Port=4
  wires:
  Product3/1 -> Subtract/2
  Product2/1 -> Subtract/1
  Add1/1 -> Id/1  "Id"
  Subtract/1 -> Iq/1  "Iq"
  Product/1 -> Add1/1
  Product1/1 -> Add1/2
  CosTheta/1 -> Product3/2, Product/2
  SinTheta/1 -> Product2/2, Product1/2
  a_plus_2b/1 -> one_by_sqrt3/1
  one_by_sqrt3/1 -> Ibeta/1, Product3/1, Product1/1  "Ibeta"
  Signal Copy/1 -> Ialpha/1, Product2/1, Product/1  "Ialpha"
  Ia/1 -> a_plus_2b/1, Signal Copy/1
  Ib/1 -> a_plus_2b/3, a_plus_2b/2
